simulink model "black_scholes_model"  (R2021a)
settings: Solver=VariableStepAuto  StartTime=0.0  StopTime=10.0  RelTol=1e-3
settings Model: Creator=jonas  LastModifiedBy=jonas

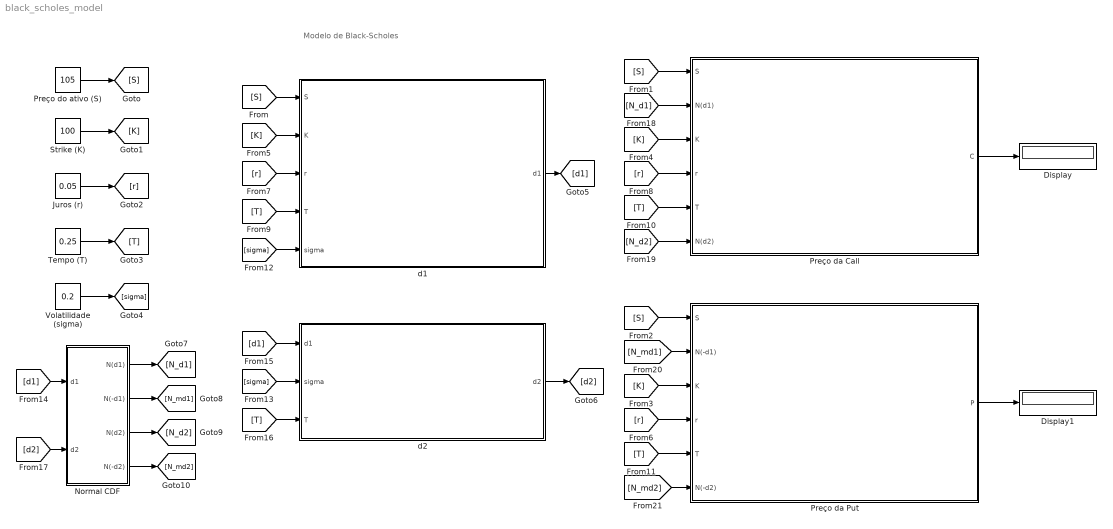
== system black_scholes_model ==
  note: Modelo de Black-Scholes
  Display : Display
  Display1 : Display
  Juros (r) : Constant  Value=0.05
  Normal CDF : Subsystem
  Preço da Call : Subsystem
  Preço da Put : Subsystem
  Preço do ativo (S) : Constant  Value=105
  Strike (K) : Constant  Value=100
  Tempo (T) : Constant  Value=0.25
  Volatilidade (sigma) : Constant  Value=0.2
  d1 : Subsystem
  d2 : Subsystem
  wires:
  Preço do ativo (S)/1 -> [S]
  Strike (K)/1 -> [K]
  Juros (r)/1 -> [r]
  Tempo (T)/1 -> [T]
  Volatilidade (sigma)/1 -> [sigma]
  d1/1(d1) -> [d1]
  d2/1(d2) -> [d2]
  [S] -> d1/1(S)
  [S] -> Preço da Call/1(S)
  [S] -> Preço da Put/1(S)
  [K] -> d1/2(K)
  [K] -> Preço da Call/3(K)
  [K] -> Preço da Put/3(K)
  [r] -> d1/3(r)
  [r] -> Preço da Call/4(r)
  [r] -> Preço da Put/4(r)
  [T] -> d1/4(T)
  [T] -> Preço da Call/5(T)
  [T] -> Preço da Put/5(T)
  [sigma] -> d2/2(sigma)
  [sigma] -> d1/5(sigma)
  [d1] -> d2/1(d1)
  [d1] -> Normal CDF/1(d1)
  [T] -> d2/3(T)
  [d2] -> Normal CDF/2(d2)
  Normal CDF/1(N(d1)) -> [N_d1]
  Normal CDF/2(N(-d1)) -> [N_md1]
  Normal CDF/3(N(d2)) -> [N_d2]
  Normal CDF/4(N(-d2)) -> [N_md2]
  [N_d1] -> Preço da Call/2(N(d1))
  [N_d2] -> Preço da Call/6(N(d2))
  [N_md1] -> Preço da Put/2(N(-d1))
  [N_md2] -> Preço da Put/6(N(-d2))
  Preço da Call/1(C) -> Display/1
  Preço da Put/1(P) -> Display1/1

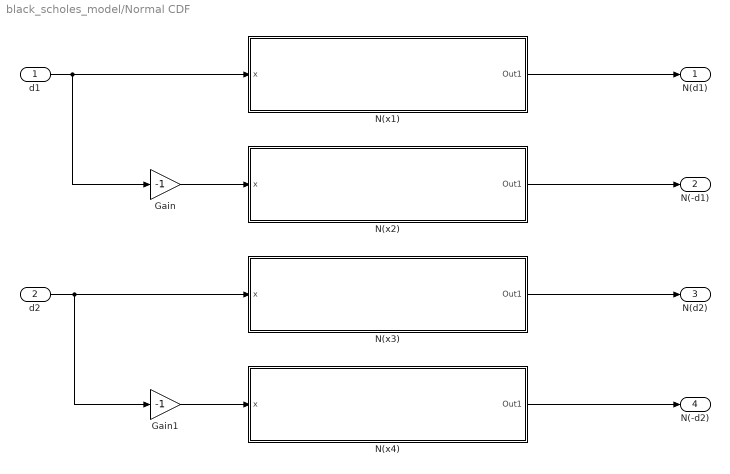
== system black_scholes_model/Normal CDF ==
  d1 : Inport
  d2 : Inport  Port=2
  Gain : Gain  Gain=-1
  Gain1 : Gain  Gain=-1
  N(x1) : Subsystem
  N(x2) : Subsystem
  N(x3) : Subsystem
  N(x4) : Subsystem
  N(d1) : Outport
  N(-d1) : Outport  Port=2
  N(d2) : Outport  Port=3
  N(-d2) : Outport  Port=4
  wires:
  Gain1/1 -> N(x4)/1(x)
  Gain/1 -> N(x2)/1(x)
  d1/1 -> Gain/1, N(x1)/1(x)
  d2/1 -> Gain1/1, N(x3)/1(x)
  N(x4)/1(Out1) -> N(-d2)/1
  N(x3)/1(Out1) -> N(d2)/1
  N(x2)/1(Out1) -> N(-d1)/1
  N(x1)/1(Out1) -> N(d1)/1

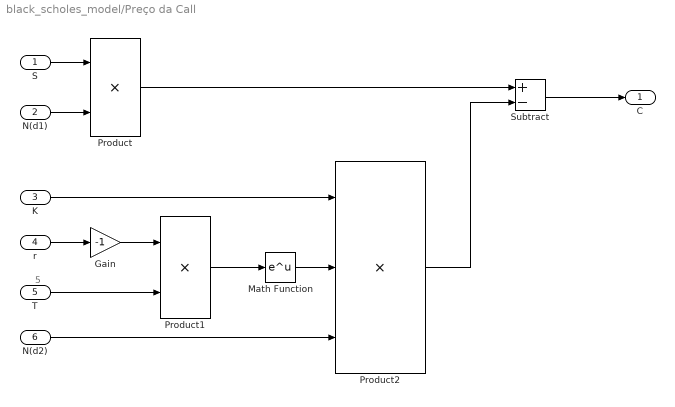
== system black_scholes_model/Preço da Call ==
  note: 5
  S : Inport
  N(d1) : Inport  Port=2
  K : Inport  Port=3
  r : Inport  Port=4
  T : Inport  Port=5
  N(d2) : Inport  Port=6
  Gain : Gain  Gain=-1
  Math Function : Math  SaturateOnIntegerOverflow=on
  Product : Product
  Product1 : Product
  Product2 : Product  Inputs=3
  Subtract : Sum  Inputs=+-
  C : Outport
  wires:
  S/1 -> Product/1
  N(d1)/1 -> Product/2
  r/1 -> Gain/1
  T/1 -> Product1/2
  Gain/1 -> Product1/1
  Product1/1 -> Math Function/1
  K/1 -> Product2/1
  Math Function/1 -> Product2/2
  N(d2)/1 -> Product2/3
  Product/1 -> Subtract/1
  Product2/1 -> Subtract/2
  Subtract/1 -> C/1

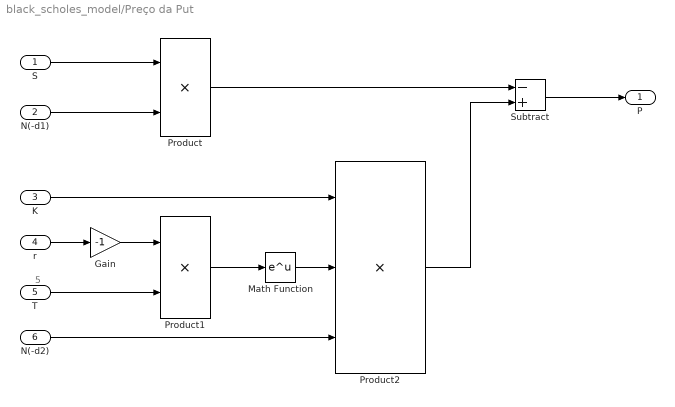
== system black_scholes_model/Preço da Put ==
  note: 5
  S : Inport
  N(-d1) : Inport  Port=2
  K : Inport  Port=3
  r : Inport  Port=4
  T : Inport  Port=5
  N(-d2) : Inport  Port=6
  Gain : Gain  Gain=-1
  Math Function : Math  SaturateOnIntegerOverflow=on
  Product : Product
  Product1 : Product
  Product2 : Product  Inputs=3
  Subtract : Sum  Inputs=-+
  P : Outport
  wires:
  S/1 -> Product/1
  N(-d1)/1 -> Product/2
  r/1 -> Gain/1
  T/1 -> Product1/2
  Gain/1 -> Product1/1
  Product1/1 -> Math Function/1
  K/1 -> Product2/1
  Math Function/1 -> Product2/2
  N(-d2)/1 -> Product2/3
  Product/1 -> Subtract/1
  Product2/1 -> Subtract/2
  Subtract/1 -> P/1

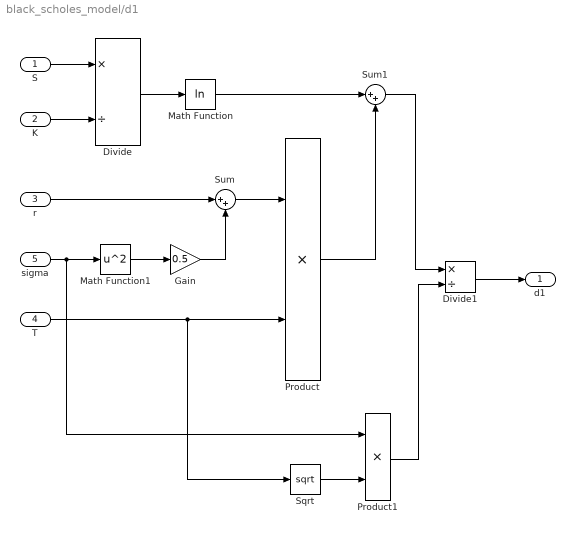
== system black_scholes_model/d1 ==
  S : Inport
  K : Inport  Port=2
  r : Inport  Port=3
  T : Inport  Port=4
  sigma : Inport  Port=5
  Divide : Product  Inputs=*/
  Divide1 : Product  Inputs=*/
  Gain : Gain  Gain=0.5
  Math Function : Math  Operator=log  SaturateOnIntegerOverflow=on
  Math Function1 : Math  Operator=square  SaturateOnIntegerOverflow=on
  Product : Product
  Product1 : Product
  Sqrt : Sqrt  SaturateOnIntegerOverflow=on
  Sum : Sum  Inputs=|++
  Sum1 : Sum  Inputs=|++
  d1 : Outport
  wires:
  K/1 -> Divide/2
  S/1 -> Divide/1
  Divide/1 -> Math Function/1
  sigma/1 -> Product1/1, Math Function1/1
  r/1 -> Sum/1
  Math Function1/1 -> Gain/1
  Gain/1 -> Sum/2
  Sum/1 -> Product/1
  T/1 -> Sqrt/1, Product/2
  Math Function/1 -> Sum1/1
  Product/1 -> Sum1/2
  Sqrt/1 -> Product1/2
  Sum1/1 -> Divide1/1
  Product1/1 -> Divide1/2
  Divide1/1 -> d1/1

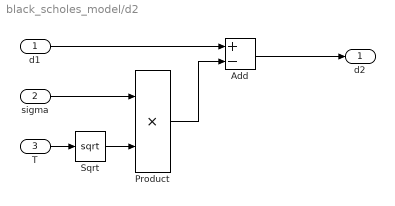
== system black_scholes_model/d2 ==
  d1 : Inport
  sigma : Inport  Port=2
  T : Inport  Port=3
  Add : Sum  Inputs=+-
  Product : Product
  Sqrt : Sqrt  SaturateOnIntegerOverflow=on
  d2 : Outport
  wires:
  T/1 -> Sqrt/1
  Sqrt/1 -> Product/2
  sigma/1 -> Product/1
  d1/1 -> Add/1
  Product/1 -> Add/2
  Add/1 -> d2/1

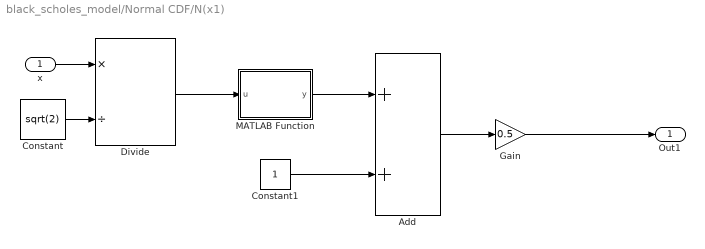
== system black_scholes_model/Normal CDF/N(x1) ==
  x : Inport
  Add : Sum
  Constant : Constant  Value=sqrt(2)
  Constant1 : Constant
  Divide : Product  Inputs=*/
  Gain : Gain  Gain=0.5
  MATLAB Function : MATLAB Function  TreatAsAtomicUnit=on
  Out1 : Outport
  wires:
  Constant/1 -> Divide/2
  x/1 -> Divide/1
  Divide/1 -> MATLAB Function/1(u)
  Constant1/1 -> Add/2
  MATLAB Function/1(y) -> Add/1
  Add/1 -> Gain/1
  Gain/1 -> Out1/1

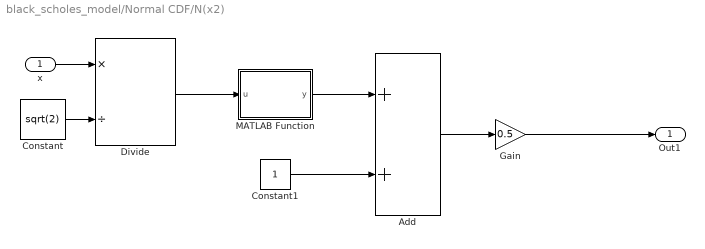
== system black_scholes_model/Normal CDF/N(x2) ==
  x : Inport
  Add : Sum
  Constant : Constant  Value=sqrt(2)
  Constant1 : Constant
  Divide : Product  Inputs=*/
  Gain : Gain  Gain=0.5
  MATLAB Function : MATLAB Function  TreatAsAtomicUnit=on
  Out1 : Outport
  wires:
  Constant/1 -> Divide/2
  x/1 -> Divide/1
  Divide/1 -> MATLAB Function/1(u)
  Constant1/1 -> Add/2
  MATLAB Function/1(y) -> Add/1
  Add/1 -> Gain/1
  Gain/1 -> Out1/1

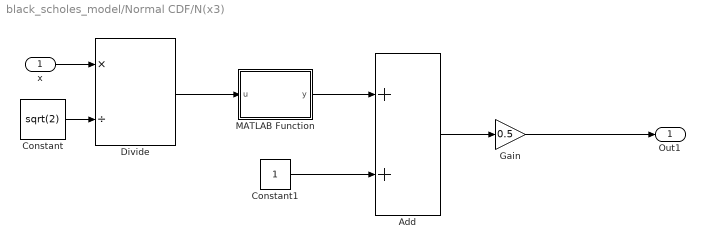
== system black_scholes_model/Normal CDF/N(x3) ==
  x : Inport
  Add : Sum
  Constant : Constant  Value=sqrt(2)
  Constant1 : Constant
  Divide : Product  Inputs=*/
  Gain : Gain  Gain=0.5
  MATLAB Function : MATLAB Function  TreatAsAtomicUnit=on
  Out1 : Outport
  wires:
  Constant/1 -> Divide/2
  x/1 -> Divide/1
  Divide/1 -> MATLAB Function/1(u)
  Constant1/1 -> Add/2
  MATLAB Function/1(y) -> Add/1
  Add/1 -> Gain/1
  Gain/1 -> Out1/1

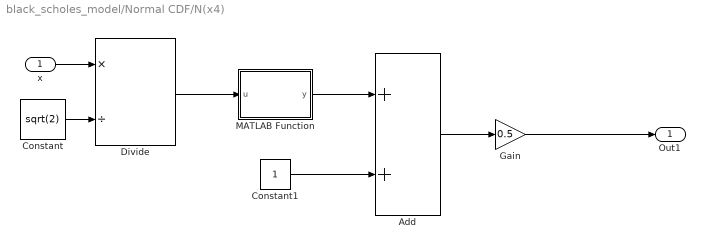
== system black_scholes_model/Normal CDF/N(x4) ==
  x : Inport
  Add : Sum
  Constant : Constant  Value=sqrt(2)
  Constant1 : Constant
  Divide : Product  Inputs=*/
  Gain : Gain  Gain=0.5
  MATLAB Function : MATLAB Function  TreatAsAtomicUnit=on
  Out1 : Outport
  wires:
  Constant/1 -> Divide/2
  x/1 -> Divide/1
  Divide/1 -> MATLAB Function/1(u)
  Constant1/1 -> Add/2
  MATLAB Function/1(y) -> Add/1
  Add/1 -> Gain/1
  Gain/1 -> Out1/1

== matlab function black_scholes_model/Normal CDF/N(x1)/MATLAB Function ==
  data: u input; y output
function y = fcn(u)
y = erf(u(1));

== matlab function black_scholes_model/Normal CDF/N(x3)/MATLAB Function ==
  data: u input; y output
function y = fcn(u)
y = erf(u(1));

== matlab function black_scholes_model/Normal CDF/N(x4)/MATLAB Function ==
  data: u input; y output
function y = fcn(u)
y = erf(u(1));

== matlab function black_scholes_model/Normal CDF/N(x2)/MATLAB Function ==
  data: u input; y output
function y = fcn(u)
y = erf(u(1));
